simulink model "gm_spectrum_analyser"  (R2020a)
settings: Solver=VariableStepAuto  StartTime=0.0  StopTime=100000/256e6  RelTol=1e-3
InitFcn:
  | fs = 256e6;
undefined symbols (not defined in the file or in its folder): designMultirateFIR
libraries: hdlsllib x81, simulink x50, dspmlti4 x6, dsphdlxfrm x5, hdlmdlgenlib x4, dspswit3 x4, dspsigops x2, dspsigattribs x2
(part 3 of 5)

== system gm_spectrum_analyser/Spectrum Analyser/Spectrum Analyser/Spectrum Analyser Core/FFT and Spectrum Processing/FFT Core ==
  Data In : Inport  OutDataTypeStr=fixdt(1, 16, 15)  PortDimensions=1  SampleTime=3.90625e-09
      settings: SignalType=complex
  Valid In : Inport  Port=2  OutDataTypeStr=boolean  PortDimensions=1  SampleTime=3.90625e-09
  Selector : Inport  Port=3  OutDataTypeStr=uint8  PortDimensions=1  SampleTime=3.90625e-09
  AND{1..5} (5 alike) : Logic  AllPortsSameDT=off  OutDataTypeStr=boolean  SampleTime=3.90625e-09
  Compare To Constant : simulink/Logic and Bit Operations/Compare To Constant  relop===  const="fi(0,0,8,0,\"hex\",\"00\")"  OutDataTypeStr=boolean
  Compare To Constant1 : simulink/Logic and Bit Operations/Compare To Constant  relop===  const="fi(0,0,8,0,\"hex\",\"01\")"  OutDataTypeStr=boolean
  Compare To Constant2 : simulink/Logic and Bit Operations/Compare To Constant  relop===  const="fi(0,0,8,0,\"hex\",\"02\")"  OutDataTypeStr=boolean
  Compare To Constant3 : simulink/Logic and Bit Operations/Compare To Constant  relop===  const="fi(0,0,8,0,\"hex\",\"03\")"  OutDataTypeStr=boolean
  Compare To Constant4 : simulink/Logic and Bit Operations/Compare To Constant  relop===  const="fi(0,0,8,0,\"hex\",\"04\")"  OutDataTypeStr=boolean
  FFT HDL Optimized 16384 : dsphdlxfrm/FFT HDL Optimized  FFTLength=16384  Architecture=Streaming Radix 2^2  ComplexMultiplication=Use 4 multipliers and 2 adders  BitReversedOutput=off  BitReversedInput=off  Normalize=off  SimulateUsing=Code generation  RoundingMethod=Round  ResetInputPort=off  StartOutputPort=on  EndOutputPort=on
      settings: SourceProductBaseCode=DS
  FFT HDL Optimized 32768 : dsphdlxfrm/FFT HDL Optimized  FFTLength=32768  Architecture=Streaming Radix 2^2  ComplexMultiplication=Use 4 multipliers and 2 adders  BitReversedOutput=off  BitReversedInput=off  Normalize=off  SimulateUsing=Code generation  RoundingMethod=Round  ResetInputPort=off  StartOutputPort=on  EndOutputPort=on
      settings: SourceProductBaseCode=DS
  FFT HDL Optimized 4096 : dsphdlxfrm/FFT HDL Optimized  FFTLength=4096  Architecture=Streaming Radix 2^2  ComplexMultiplication=Use 4 multipliers and 2 adders  BitReversedOutput=off  BitReversedInput=off  Normalize=off  SimulateUsing=Code generation  RoundingMethod=Round  ResetInputPort=off  StartOutputPort=on  EndOutputPort=on
      settings: SourceProductBaseCode=DS
  FFT HDL Optimized 65536 : dsphdlxfrm/FFT HDL Optimized  FFTLength=65536  Architecture=Streaming Radix 2^2  ComplexMultiplication=Use 4 multipliers and 2 adders  BitReversedOutput=off  BitReversedInput=off  Normalize=off  SimulateUsing=Code generation  RoundingMethod=Round  ResetInputPort=off  StartOutputPort=on  EndOutputPort=on
      settings: SourceProductBaseCode=DS
  FFT HDL Optimized 8192 : dsphdlxfrm/FFT HDL Optimized  FFTLength=8192  Architecture=Streaming Radix 2^2  ComplexMultiplication=Use 4 multipliers and 2 adders  BitReversedOutput=off  BitReversedInput=off  Normalize=off  SimulateUsing=Code generation  RoundingMethod=Round  ResetInputPort=off  StartOutputPort=on  EndOutputPort=on
      settings: SourceProductBaseCode=DS
  Multiport Switch : MultiPortSwitch  DataPortOrder=Zero-based contiguous  Inputs=5  DiagnosticForDefault=None  zeroidx=on  OutDataTypeStr=fixdt(1, 32, 15)  SampleTime=3.90625e-09
  Multiport Switch1 : MultiPortSwitch  DataPortOrder=Zero-based contiguous  Inputs=5  DiagnosticForDefault=None  zeroidx=on  SampleTime=3.90625e-09
  Multiport Switch2 : MultiPortSwitch  DataPortOrder=Zero-based contiguous  Inputs=5  DiagnosticForDefault=None  zeroidx=on  SampleTime=3.90625e-09
  Multiport Switch3 : MultiPortSwitch  DataPortOrder=Zero-based contiguous  Inputs=5  DiagnosticForDefault=None  zeroidx=on  SampleTime=3.90625e-09
  Data Out : Outport
  Start : Outport  Port=2
  End : Outport  Port=3
  Valid Out : Outport  Port=4
  wires:
  AND1/1 -> FFT HDL Optimized 4096/2
  AND2/1 -> FFT HDL Optimized 8192/2
  AND3/1 -> FFT HDL Optimized 16384/2
  AND4/1 -> FFT HDL Optimized 32768/2
  AND5/1 -> FFT HDL Optimized 65536/2
  Compare To Constant/1 -> AND1/2
  Compare To Constant1/1 -> AND2/2
  Compare To Constant2/1 -> AND3/2
  Compare To Constant3/1 -> AND4/2
  Compare To Constant4/1 -> AND5/2
  FFT HDL Optimized 16384/1 -> Multiport Switch/4
  FFT HDL Optimized 16384/2 -> Multiport Switch1/4
  FFT HDL Optimized 16384/3 -> Multiport Switch2/4
  FFT HDL Optimized 16384/4 -> Multiport Switch3/4
  FFT HDL Optimized 32768/1 -> Multiport Switch/5
  FFT HDL Optimized 32768/2 -> Multiport Switch1/5
  FFT HDL Optimized 32768/3 -> Multiport Switch2/5
  FFT HDL Optimized 32768/4 -> Multiport Switch3/5
  FFT HDL Optimized 4096/1 -> Multiport Switch/2
  FFT HDL Optimized 4096/2 -> Multiport Switch1/2
  FFT HDL Optimized 4096/3 -> Multiport Switch2/2
  FFT HDL Optimized 4096/4 -> Multiport Switch3/2
  FFT HDL Optimized 65536/1 -> Multiport Switch/6
  FFT HDL Optimized 65536/2 -> Multiport Switch1/6
  FFT HDL Optimized 65536/3 -> Multiport Switch2/6
  FFT HDL Optimized 65536/4 -> Multiport Switch3/6
  FFT HDL Optimized 8192/1 -> Multiport Switch/3
  FFT HDL Optimized 8192/2 -> Multiport Switch1/3
  FFT HDL Optimized 8192/3 -> Multiport Switch2/3
  FFT HDL Optimized 8192/4 -> Multiport Switch3/3
  Multiport Switch/1 -> Data Out/1
  Multiport Switch1/1 -> Start/1
  Multiport Switch2/1 -> End/1
  Multiport Switch3/1 -> Valid Out/1
  Data In/1 -> FFT HDL Optimized 16384/1, FFT HDL Optimized 32768/1, FFT HDL Optimized 4096/1, FFT HDL Optimized 65536/1, FFT HDL Optimized 8192/1
  Valid In/1 -> AND5/1, AND4/1, AND3/1, AND2/1, AND1/1
  Selector/1 -> Multiport Switch3/1, Multiport Switch2/1, Multiport Switch1/1, Multiport Switch/1, Compare To Constant4/1, Compare To Constant3/1, Compare To Constant2/1, Compare To Constant1/1, Compare To Constant/1

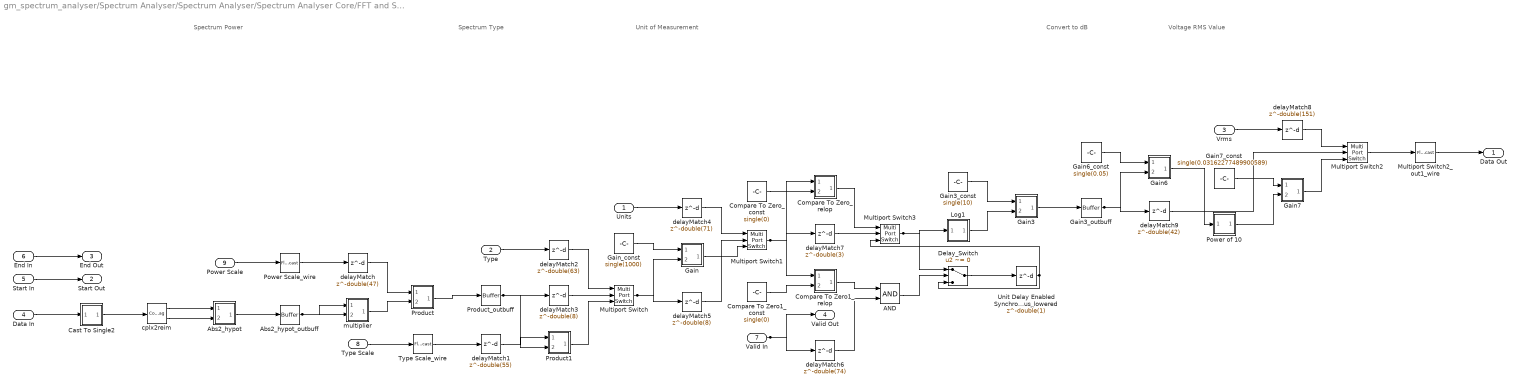
== system gm_spectrum_analyser/Spectrum Analyser/Spectrum Analyser/Spectrum Analyser Core/FFT and Spectrum Processing/Spectrum Options ==
  note: Voltage RMS Value
  note: Convert to dB
  note: Unit of Measurement
  note: Spectrum Type
  note: Spectrum Power
  Units : Inport  OutDataTypeStr=uint32  PortDimensions=1  SampleTime=3.90625e-09
  Type : Inport  Port=2  OutDataTypeStr=uint32  PortDimensions=1  SampleTime=3.90625e-09
  Vrms : Inport  Port=3  OutDataTypeStr=uint32  PortDimensions=1  SampleTime=3.90625e-09
  Data In : Inport  Port=4  OutDataTypeStr=fixdt(1, 32, 15)  PortDimensions=1  SampleTime=3.90625e-09
      settings: SignalType=complex
  Start In : Inport  Port=5  OutDataTypeStr=boolean  PortDimensions=1  SampleTime=3.90625e-09
  End In : Inport  Port=6  OutDataTypeStr=boolean  PortDimensions=1  SampleTime=3.90625e-09
  Valid In : Inport  Port=7  OutDataTypeStr=boolean  PortDimensions=1  SampleTime=3.90625e-09
  Type Scale : Inport  Port=8  OutDataTypeStr=uint32  PortDimensions=1  SampleTime=3.90625e-09
  Power Scale : Inport  Port=9  OutDataTypeStr=uint32  PortDimensions=1  SampleTime=3.90625e-09
  AND : Logic  AllPortsSameDT=off  OutDataTypeStr=boolean  SampleTime=3.90625e-09
  Abs2_hypot : Subsystem
      mask Display: disp('NFP\nmath2');
  Abs2_hypot_outbuff : hdlmdlgenlib/Buffer
      settings: SourceProductBaseCode=SL
  Cast To Single2 : Subsystem
      mask Display: disp('NFP\nconv');
  Compare To Zero1_const : Constant  Value=single(0)  OutDataTypeStr=single  SampleTime=3.90625e-09
  Compare To Zero1_relop : Subsystem
      mask Display: disp('NFP\nrelop');
  Compare To Zero_const : Constant  Value=single(0)  OutDataTypeStr=single  SampleTime=3.90625e-09
  Compare To Zero_relop : Subsystem
      mask Display: disp('NFP\nrelop');
  Delay_Switch : Switch  Criteria=u2 ~= 0  Threshold=double(0)  OutDataTypeStr=single  SampleTime=3.90625e-09
  Gain : Subsystem
      mask Display: disp('NFP\nmul');
  Gain3 : Subsystem
      mask Display: disp('NFP\nmul');
  Gain3_const : Constant  Value=single(10)  OutDataTypeStr=single  SampleTime=3.90625e-09
  Gain3_outbuff : hdlmdlgenlib/Buffer
      settings: SourceProductBaseCode=SL
  Gain6 : Subsystem
      mask Display: disp('NFP\nmul');
  Gain6_const : Constant  Value=single(0.05)  OutDataTypeStr=single  SampleTime=3.90625e-09
  Gain7 : Subsystem
      mask Display: disp('NFP\nmul');
  Gain7_const : Constant  Value=single(0.03162277489900589)  OutDataTypeStr=single  SampleTime=3.90625e-09
  Gain_const : Constant  Value=single(1000)  OutDataTypeStr=single  SampleTime=3.90625e-09
  Log1 : Subsystem
      mask Display: disp('NFP\nmath');
  Multiport Switch{,1..3} (4 alike) : MultiPortSwitch  DataPortOrder=Zero-based contiguous  Inputs=2  DiagnosticForDefault=None  zeroidx=on  OutDataTypeStr=single  SampleTime=3.90625e-09
  Multiport Switch2_out1_wire : FloatTypecast
  Power Scale_wire : FloatTypecast
  Power of 10 : Subsystem
      mask Display: disp('NFP\nmath');
  Product : Subsystem
      mask Display: disp('NFP\nmul');
  Product1 : Subsystem
      mask Display: disp('NFP\nmul');
  Product_outbuff : hdlmdlgenlib/Buffer
      settings: SourceProductBaseCode=SL
  Type Scale_wire : FloatTypecast
  Unit Delay Enabled Synchronous_lowered : Delay  DelayLength=double(1)  InitialCondition=0  SampleTime=3.90625e-09
  cplx2reim : ComplexToRealImag  SampleTime=3.90625e-09
  delayMatch : Delay  DelayLength=double(47)  InitialCondition=0  SampleTime=3.90625e-09
  delayMatch1 : Delay  DelayLength=double(55)  InitialCondition=0  SampleTime=3.90625e-09
  delayMatch2 : Delay  DelayLength=double(63)  InitialCondition=0  SampleTime=3.90625e-09
  delayMatch3 : Delay  DelayLength=double(8)  InitialCondition=0  SampleTime=3.90625e-09
  delayMatch4 : Delay  DelayLength=double(71)  InitialCondition=0  SampleTime=3.90625e-09
  delayMatch5 : Delay  DelayLength=double(8)  InitialCondition=0  SampleTime=3.90625e-09
  delayMatch6 : Delay  DelayLength=double(74)  InitialCondition=0  SampleTime=3.90625e-09
  delayMatch7 : Delay  DelayLength=double(3)  InitialCondition=0  SampleTime=3.90625e-09
  delayMatch8 : Delay  DelayLength=double(151)  InitialCondition=0  SampleTime=3.90625e-09
  delayMatch9 : Delay  DelayLength=double(42)  InitialCondition=0  SampleTime=3.90625e-09
  multiplier : Subsystem
      mask Display: disp('NFP\nmul');
  Data Out : Outport
  Start Out : Outport  Port=2
  End Out : Outport  Port=3
  Valid Out : Outport  Port=4
  wires:
  AND/1 -> Delay_Switch/2
  Abs2_hypot_outbuff/1 -> multiplier/2(In2), multiplier/1(In1)
  Multiport Switch2_out1_wire/1 -> Data Out/1
  delayMatch1/1 -> Product1/1(In1)
  delayMatch/1 -> Product/1(In1)
  delayMatch9/1 -> Multiport Switch2/2
  delayMatch5/1 -> Multiport Switch1/2
  delayMatch7/1 -> Multiport Switch3/2
  Multiport Switch2/1 -> Multiport Switch2_out1_wire/1
  delayMatch3/1 -> Multiport Switch/2
  cplx2reim/1 -> Abs2_hypot/1(In1)
  cplx2reim/2 -> Abs2_hypot/2(In2)
  Compare To Zero_const/1 -> Compare To Zero_relop/2(In2)
  Compare To Zero1_const/1 -> Compare To Zero1_relop/2(In2)
  Gain_const/1 -> Gain/1(In1)
  Gain3_const/1 -> Gain3/1(In1)
  Gain6_const/1 -> Gain6/1(In1)
  Gain7_const/1 -> Gain7/1(In1)
  delayMatch4/1 -> Multiport Switch1/1
  delayMatch2/1 -> Multiport Switch/1
  delayMatch8/1 -> Multiport Switch2/1
  delayMatch6/1 -> AND/2
  Abs2_hypot/1(Out1) -> Abs2_hypot_outbuff/1
  Cast To Single2/1(Out1) -> cplx2reim/1
  Compare To Zero_relop/1(Out1) -> Multiport Switch3/1
  Compare To Zero1_relop/1(Out1) -> AND/1
  Log1/1(Out1) -> Gain3/2(In2)
  Power of 10/1(Out1) -> Gain7/2(In2)
  Product/1(Out1) -> Product_outbuff/1
  Product1/1(Out1) -> Multiport Switch/3
  multiplier/1(Out1) -> Product/2(In2)
  Gain/1(Out1) -> Multiport Switch1/3
  Gain3/1(Out1) -> Gain3_outbuff/1
  Gain6/1(Out1) -> Power of 10/1(In1)
  Gain7/1(Out1) -> Multiport Switch2/3
  Power Scale_wire/1 -> delayMatch/1
  Type Scale_wire/1 -> delayMatch1/1
  Product_outbuff/1 -> delayMatch3/1, Product1/2(In2)
  Multiport Switch/1 -> delayMatch5/1, Gain/2(In2)
  Multiport Switch1/1 -> delayMatch7/1, Compare To Zero1_relop/1(In1), Compare To Zero_relop/1(In1)
  Gain3_outbuff/1 -> delayMatch9/1, Gain6/2(In2)
  Multiport Switch3/1 -> Log1/1(In1), Delay_Switch/1
  Units/1 -> delayMatch4/1
  Type/1 -> delayMatch2/1
  Vrms/1 -> delayMatch8/1
  Data In/1 -> Cast To Single2/1(In1)
  Start In/1 -> Start Out/1
  End In/1 -> End Out/1
  Valid In/1 -> delayMatch6/1, Valid Out/1
  Type Scale/1 -> Type Scale_wire/1
  Power Scale/1 -> Power Scale_wire/1
  Delay_Switch/1 -> Unit Delay Enabled Synchronous_lowered/1
  Unit Delay Enabled Synchronous_lowered/1 -> Multiport Switch3/3, Delay_Switch/3

== system gm_spectrum_analyser/Spectrum Analyser/Spectrum Analyser/Spectrum Analyser Core/Preprocessing Window/Direct Memory Access ==
  axim_rd_s2m : Inport  SampleTime=3.90625e-09
  axim_rd_data : Inport  Port=2  OutDataTypeStr=uint16  PortDimensions=1  SampleTime=3.90625e-09
  Length : Inport  Port=3  OutDataTypeStr=uint32  PortDimensions=1  SampleTime=3.90625e-09
  Address : Inport  Port=4  OutDataTypeStr=uint32  PortDimensions=1  SampleTime=3.90625e-09
  Enable DMA : Inport  Port=5  OutDataTypeStr=uint32  PortDimensions=1  SampleTime=3.90625e-09
  Bit Slice : hdlsllib/Logic and Bit Operations/Bit Slice  lidx=double(0)  ridx=double(0)
      settings: SourceProductBaseCode=SL
  Bus Creator : BusCreator  Inputs=3
  DDR Read Controller : Subsystem
  EdgeDetection : Subsystem
  bus_selector : BusSelector  OutputSignals=rd_aready,rd_dvalid
  ram_wr_data : Outport  VectorParamsAs1DForOutWhenUnconnected=off
  ram_wr_addr : Outport  Port=2  VectorParamsAs1DForOutWhenUnconnected=off
  ram_wren : Outport  Port=3  VectorParamsAs1DForOutWhenUnconnected=off
  dma_read_ready : Outport  Port=4  VectorParamsAs1DForOutWhenUnconnected=off
  axim_rd_m2s : Outport  Port=5  VectorParamsAs1DForOutWhenUnconnected=off
  wires:
  Bit Slice/1 -> EdgeDetection/1(In1)
  Bus Creator/1 -> axim_rd_m2s/1
  bus_selector/1 -> DDR Read Controller/4(rd_aready)  "<rd_aready>"
  bus_selector/2 -> DDR Read Controller/5(rd_dvalid)  "<rd_dvalid>"
  DDR Read Controller/1(valid_out) -> ram_wren/1
  DDR Read Controller/2(count_out) -> ram_wr_addr/1
  DDR Read Controller/3(ready_out) -> dma_read_ready/1
  DDR Read Controller/4(rd_addr) -> Bus Creator/1  "rd_addr"
  DDR Read Controller/5(rd_len) -> Bus Creator/2  "rd_len"
  DDR Read Controller/6(rd_avalid) -> Bus Creator/3  "rd_avalid"
  EdgeDetection/1(Out1) -> DDR Read Controller/3(start)
  axim_rd_s2m/1 -> bus_selector/1
  axim_rd_data/1 -> ram_wr_data/1
  Length/1 -> DDR Read Controller/1(length_in)
  Address/1 -> DDR Read Controller/2(address)
  Enable DMA/1 -> Bit Slice/1

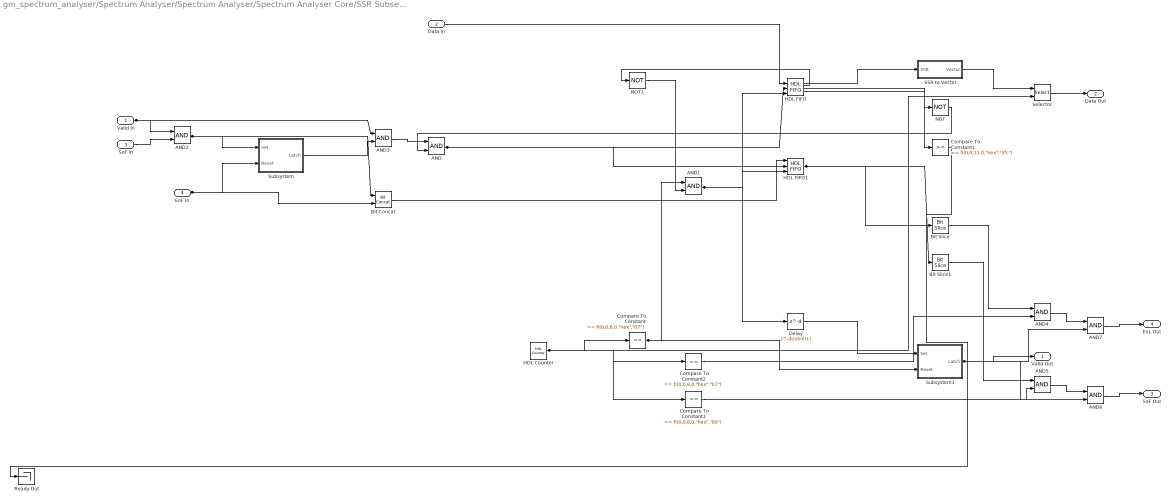
== system gm_spectrum_analyser/Spectrum Analyser/Spectrum Analyser/Spectrum Analyser Core/SSR Subset Converter/SSR Deserializer Imag ==
  Valid In : Inport  OutDataTypeStr=boolean  PortDimensions=1  SampleTime=3.90625e-09
  Data In : Inport  Port=2  OutDataTypeStr=fixdt(0, 128, 0)  PortDimensions=1  SampleTime=3.90625e-09
  SoF In : Inport  Port=3  OutDataTypeStr=boolean  PortDimensions=1  SampleTime=3.90625e-09
  EoF In : Inport  Port=4  OutDataTypeStr=boolean  PortDimensions=1  SampleTime=3.90625e-09
  AND{,1..7} (8 alike) : Logic  AllPortsSameDT=off  OutDataTypeStr=boolean  SampleTime=3.90625e-09
  Bit Concat : hdlsllib/Logic and Bit Operations/Bit Concat  numInputs=2
  Bit Slice : hdlsllib/Logic and Bit Operations/Bit Slice  lidx=double(0)  ridx=double(0)
      settings: SourceProductBaseCode=SL
  Bit Slice1 : hdlsllib/Logic and Bit Operations/Bit Slice  lidx=double(1)  ridx=double(1)
      settings: SourceProductBaseCode=SL
  Compare To Constant : simulink/Logic and Bit Operations/Compare To Constant  relop===  const="fi(0,0,8,0,\"hex\",\"07\")"  OutDataTypeStr=boolean
  Compare To Constant1 : simulink/Logic and Bit Operations/Compare To Constant  relop=>=  const="fi(0,0,11,0,\"hex\",\"3fc\")"  OutDataTypeStr=boolean
  Compare To Constant2 : simulink/Logic and Bit Operations/Compare To Constant  relop===  const="fi(0,0,8,0,\"hex\",\"07\")"  OutDataTypeStr=boolean
  Compare To Constant3 : simulink/Logic and Bit Operations/Compare To Constant  relop===  const="fi(0,0,8,0,\"hex\",\"00\")"  OutDataTypeStr=boolean
  Delay : Delay  DelayLength=double(1)  InitialCondition=0  SampleTime=3.90625e-09
  HDL Counter : hdlsllib/Sources/HDL Counter  CountType=Count limited  CountInit=double(0)  CountStep=double(1)  CountMax=double(7)  CountFromType=Initial value  CountFrom=double(0)  CountResetPort=off  CountLoadPort=off  CountEnbPort=off  CountDirPort=off  CountDataType=Unsigned  CountWordLen=8  CountFracLen=0  CountSampTime=3.90625e-09
  HDL FIFO : hdlsllib/HDL RAMs/HDL FIFO  fifo_size=1024  mode=Classic  ratio=1  push_msg=Error  pop_msg=Error  show_empty=on  show_full=on  show_num=on  LabelModeActiveChoice_Mode=Classic
      settings: SourceProductBaseCode=SL
  HDL FIFO1 : hdlsllib/HDL RAMs/HDL FIFO  fifo_size=1024  mode=Classic  ratio=1  push_msg=Error  pop_msg=Error  show_empty=off  show_full=off  show_num=off  LabelModeActiveChoice_Mode=Classic
      settings: SourceProductBaseCode=SL
  NOT : Logic  Operator=NOT  Inputs=1  AllPortsSameDT=off  OutDataTypeStr=boolean  SampleTime=3.90625e-09
  NOT1 : Logic  Operator=NOT  Inputs=1  AllPortsSameDT=off  OutDataTypeStr=boolean  SampleTime=3.90625e-09
  Ready Out : Terminator
  SSR to Vector : Subsystem  mask{N=double(8), w=double(16), hN=8, hw=16}
      mask prompts: N "Samples per clock cycle:"; w "Wordlength:"
  Selector : Selector  IndexMode=Zero-based  SampleTime=3.90625e-09  IndexOptions=Index vector (port)  Indices=double([1 3])  OutputSizes=double(1)
  Subsystem : Subsystem
  Subsystem1 : Subsystem
  Valid Out : Outport
  Data Out : Outport  Port=2
  SoF Out : Outport  Port=3
  EoL Out : Outport  Port=4
  wires:
  AND/1 -> HDL FIFO1/2, HDL FIFO/2
  AND1/1 -> Delay/1, HDL FIFO1/3, HDL FIFO/3
  AND2/1 -> Bit Concat/1, Subsystem/1(Set)
  AND3/1 -> AND/1
  AND4/1 -> AND7/1
  AND5/1 -> AND6/1
  AND6/1 -> SoF Out/1
  AND7/1 -> EoL Out/1
  Bit Concat/1 -> HDL FIFO1/1
  Bit Slice/1 -> AND4/1
  Bit Slice1/1 -> AND5/1
  Compare To Constant/1 -> Subsystem1/2(Reset), AND1/1
  Compare To Constant1/1 -> Ready Out/1
  Compare To Constant2/1 -> AND4/2
  Compare To Constant3/1 -> AND5/2
  Delay/1 -> Subsystem1/1(Set)
  HDL Counter/1 -> Selector/2, Compare To Constant3/1, Compare To Constant2/1, Compare To Constant/1
  HDL FIFO/1 -> SSR to Vector/1(SSR)
  HDL FIFO/4 -> Compare To Constant1/1
  HDL FIFO1/1 -> Bit Slice1/1, Bit Slice/1
  SSR to Vector/1(Vector) -> Selector/1
  Selector/1 -> Data Out/1
  Subsystem/1(Latch) -> AND3/2
  Subsystem1/1(Latch) -> AND7/2, AND6/2, Valid Out/1
  Valid In/1 -> AND3/1, AND2/1
  Data In/1 -> HDL FIFO/1
  SoF In/1 -> AND2/2
  EoF In/1 -> Bit Concat/2, Subsystem/2(Reset)
  NOT/1 -> AND/2
  HDL FIFO/2 -> NOT1/1
  HDL FIFO/3 -> NOT/1
  NOT1/1 -> AND1/2

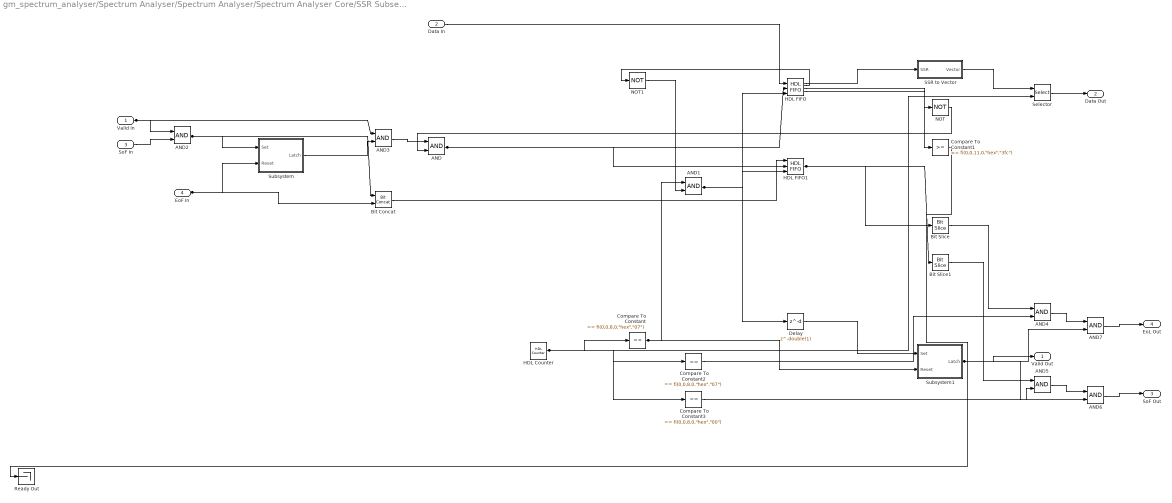
== system gm_spectrum_analyser/Spectrum Analyser/Spectrum Analyser/Spectrum Analyser Core/SSR Subset Converter/SSR Deserializer Real ==
  Valid In : Inport  OutDataTypeStr=boolean  PortDimensions=1  SampleTime=3.90625e-09
  Data In : Inport  Port=2  OutDataTypeStr=fixdt(0, 128, 0)  PortDimensions=1  SampleTime=3.90625e-09
  SoF In : Inport  Port=3  OutDataTypeStr=boolean  PortDimensions=1  SampleTime=3.90625e-09
  EoF In : Inport  Port=4  OutDataTypeStr=boolean  PortDimensions=1  SampleTime=3.90625e-09
  AND{,1..7} (8 alike) : Logic  AllPortsSameDT=off  OutDataTypeStr=boolean  SampleTime=3.90625e-09
  Bit Concat : hdlsllib/Logic and Bit Operations/Bit Concat  numInputs=2
  Bit Slice : hdlsllib/Logic and Bit Operations/Bit Slice  lidx=double(0)  ridx=double(0)
      settings: SourceProductBaseCode=SL
  Bit Slice1 : hdlsllib/Logic and Bit Operations/Bit Slice  lidx=double(1)  ridx=double(1)
      settings: SourceProductBaseCode=SL
  Compare To Constant : simulink/Logic and Bit Operations/Compare To Constant  relop===  const="fi(0,0,8,0,\"hex\",\"07\")"  OutDataTypeStr=boolean
  Compare To Constant1 : simulink/Logic and Bit Operations/Compare To Constant  relop=>=  const="fi(0,0,11,0,\"hex\",\"3fc\")"  OutDataTypeStr=boolean
  Compare To Constant2 : simulink/Logic and Bit Operations/Compare To Constant  relop===  const="fi(0,0,8,0,\"hex\",\"07\")"  OutDataTypeStr=boolean
  Compare To Constant3 : simulink/Logic and Bit Operations/Compare To Constant  relop===  const="fi(0,0,8,0,\"hex\",\"00\")"  OutDataTypeStr=boolean
  Delay : Delay  DelayLength=double(1)  InitialCondition=0  SampleTime=3.90625e-09
  HDL Counter : hdlsllib/Sources/HDL Counter  CountType=Count limited  CountInit=double(0)  CountStep=double(1)  CountMax=double(7)  CountFromType=Initial value  CountFrom=double(0)  CountResetPort=off  CountLoadPort=off  CountEnbPort=off  CountDirPort=off  CountDataType=Unsigned  CountWordLen=8  CountFracLen=0  CountSampTime=3.90625e-09
  HDL FIFO : hdlsllib/HDL RAMs/HDL FIFO  fifo_size=1024  mode=Classic  ratio=1  push_msg=Error  pop_msg=Error  show_empty=on  show_full=on  show_num=on  LabelModeActiveChoice_Mode=Classic
      settings: SourceProductBaseCode=SL
  HDL FIFO1 : hdlsllib/HDL RAMs/HDL FIFO  fifo_size=1024  mode=Classic  ratio=1  push_msg=Error  pop_msg=Error  show_empty=off  show_full=off  show_num=off  LabelModeActiveChoice_Mode=Classic
      settings: SourceProductBaseCode=SL
  NOT : Logic  Operator=NOT  Inputs=1  AllPortsSameDT=off  OutDataTypeStr=boolean  SampleTime=3.90625e-09
  NOT1 : Logic  Operator=NOT  Inputs=1  AllPortsSameDT=off  OutDataTypeStr=boolean  SampleTime=3.90625e-09
  Ready Out : Terminator
  SSR to Vector : Subsystem  mask{N=double(8), w=double(16), hN=8, hw=16}
      mask prompts: N "Samples per clock cycle:"; w "Wordlength:"
  Selector : Selector  IndexMode=Zero-based  SampleTime=3.90625e-09  IndexOptions=Index vector (port)  Indices=double([1 3])  OutputSizes=double(1)
  Subsystem : Subsystem
  Subsystem1 : Subsystem
  Valid Out : Outport
  Data Out : Outport  Port=2
  SoF Out : Outport  Port=3
  EoL Out : Outport  Port=4
  wires:
  AND/1 -> HDL FIFO1/2, HDL FIFO/2
  AND1/1 -> Delay/1, HDL FIFO1/3, HDL FIFO/3
  AND2/1 -> Bit Concat/1, Subsystem/1(Set)
  AND3/1 -> AND/1
  AND4/1 -> AND7/1
  AND5/1 -> AND6/1
  AND6/1 -> SoF Out/1
  AND7/1 -> EoL Out/1
  Bit Concat/1 -> HDL FIFO1/1
  Bit Slice/1 -> AND4/1
  Bit Slice1/1 -> AND5/1
  Compare To Constant/1 -> Subsystem1/2(Reset), AND1/1
  Compare To Constant1/1 -> Ready Out/1
  Compare To Constant2/1 -> AND4/2
  Compare To Constant3/1 -> AND5/2
  Delay/1 -> Subsystem1/1(Set)
  HDL Counter/1 -> Selector/2, Compare To Constant3/1, Compare To Constant2/1, Compare To Constant/1
  HDL FIFO/1 -> SSR to Vector/1(SSR)
  HDL FIFO/4 -> Compare To Constant1/1
  HDL FIFO1/1 -> Bit Slice1/1, Bit Slice/1
  SSR to Vector/1(Vector) -> Selector/1
  Selector/1 -> Data Out/1
  Subsystem/1(Latch) -> AND3/2
  Subsystem1/1(Latch) -> AND7/2, AND6/2, Valid Out/1
  Valid In/1 -> AND3/1, AND2/1
  Data In/1 -> HDL FIFO/1
  SoF In/1 -> AND2/2
  EoF In/1 -> Bit Concat/2, Subsystem/2(Reset)
  NOT/1 -> AND/2
  HDL FIFO/2 -> NOT1/1
  HDL FIFO/3 -> NOT/1
  NOT1/1 -> AND1/2

== system gm_spectrum_analyser/Spectrum Analyser/Spectrum Analyser/Spectrum Analyser Core/SSR Subset Converter/SSR Packet Generator Imag ==
  Frame Drop : Inport  OutDataTypeStr=fixdt(0, 4, 0)  PortDimensions=1  SampleTime=3.90625e-09
  Valid In : Inport  Port=2  OutDataTypeStr=boolean  PortDimensions=1  SampleTime=3.90625e-09
  Data In : Inport  Port=3  OutDataTypeStr=fixdt(0, 128, 0)  PortDimensions=1  SampleTime=3.90625e-09
  Packet Size : Inport  Port=4  OutDataTypeStr=uint32  PortDimensions=1  SampleTime=3.90625e-09
  Frame Dropper : Subsystem
  TLAST Generator : Subsystem
  Valid Out : Outport
  Data Out : Outport  Port=2
  SoF Out : Outport  Port=3
  EoF Out : Outport  Port=4
  wires:
  Frame Dropper/1(Valid Out) -> Valid Out/1
  Frame Dropper/2(Data Out) -> Data Out/1
  Frame Dropper/3(SoF Out) -> SoF Out/1
  Frame Dropper/4(EoF Out) -> EoF Out/1
  TLAST Generator/1(Valid Out) -> Frame Dropper/1(Valid In)
  TLAST Generator/2(Data Out) -> Frame Dropper/2(Data In)
  TLAST Generator/3(SoF Out) -> Frame Dropper/3(SoF In)
  TLAST Generator/4(EoF Out) -> Frame Dropper/4(EoF In)
  Frame Drop/1 -> Frame Dropper/5(Frame Drop)
  Valid In/1 -> TLAST Generator/1(Valid In)
  Data In/1 -> TLAST Generator/2(Data In)
  Packet Size/1 -> TLAST Generator/3(Packet Size)

== system gm_spectrum_analyser/Spectrum Analyser/Spectrum Analyser/Spectrum Analyser Core/SSR Subset Converter/SSR Packet Generator Real ==
  Frame Drop : Inport  OutDataTypeStr=fixdt(0, 4, 0)  PortDimensions=1  SampleTime=3.90625e-09
  Valid In : Inport  Port=2  OutDataTypeStr=boolean  PortDimensions=1  SampleTime=3.90625e-09
  Data In : Inport  Port=3  OutDataTypeStr=fixdt(0, 128, 0)  PortDimensions=1  SampleTime=3.90625e-09
  Packet Size : Inport  Port=4  OutDataTypeStr=uint32  PortDimensions=1  SampleTime=3.90625e-09
  Frame Dropper : Subsystem
  TLAST Generator : Subsystem
  Valid Out : Outport
  Data Out : Outport  Port=2
  SoF Out : Outport  Port=3
  EoF Out : Outport  Port=4
  wires:
  Frame Dropper/1(Valid Out) -> Valid Out/1
  Frame Dropper/2(Data Out) -> Data Out/1
  Frame Dropper/3(SoF Out) -> SoF Out/1
  Frame Dropper/4(EoF Out) -> EoF Out/1
  TLAST Generator/1(Valid Out) -> Frame Dropper/1(Valid In)
  TLAST Generator/2(Data Out) -> Frame Dropper/2(Data In)
  TLAST Generator/3(SoF Out) -> Frame Dropper/3(SoF In)
  TLAST Generator/4(EoF Out) -> Frame Dropper/4(EoF In)
  Frame Drop/1 -> Frame Dropper/5(Frame Drop)
  Valid In/1 -> TLAST Generator/1(Valid In)
  Data In/1 -> TLAST Generator/2(Data In)
  Packet Size/1 -> TLAST Generator/3(Packet Size)

== system gm_spectrum_analyser/Spectrum Analyser/Spectrum Analyser/Spectrum Analyser Core/SSR Subset Converter/SSR Serializer Imag ==
  SSR Control : Inport  OutDataTypeStr=fixdt(0, 4, 0)  PortDimensions=1  SampleTime=3.90625e-09
  Valid In : Inport  Port=2  OutDataTypeStr=boolean  PortDimensions=1  SampleTime=3.90625e-09
  Data In : Inport  Port=3  OutDataTypeStr=fixdt(0, 128, 0)  PortDimensions=1  SampleTime=3.90625e-09
  Bit Slice : hdlsllib/Logic and Bit Operations/Bit Slice  lidx=double(0)  ridx=double(0)
      settings: SourceProductBaseCode=SL
  Bit Slice1 : hdlsllib/Logic and Bit Operations/Bit Slice  lidx=double(1)  ridx=double(0)
      settings: SourceProductBaseCode=SL
  Delay : Delay  DelayLength=double(1)  InitialCondition=0  SampleTime=3.90625e-09
  Delay_Switch : Switch  Criteria=u2 ~= 0  Threshold=double(0)  OutDataTypeStr=uint16  SampleTime=3.90625e-09
  HDL Counter : hdlsllib/Sources/HDL Counter  CountType=Count limited  CountInit=double(0)  CountStep=double(1)  CountMax=double(7)  CountFromType=Initial value  CountFrom=double(0)  CountResetPort=off  CountLoadPort=off  CountEnbPort=on  CountDirPort=off  CountDataType=Unsigned  CountWordLen=3  CountFracLen=0  CountSampTime=3.90625e-09
  Multiport Switch : MultiPortSwitch  DataPortOrder=Zero-based contiguous  Inputs=4  DiagnosticForDefault=None  zeroidx=on  OutDataTypeStr=uint16  SampleTime=3.90625e-09
  Multiport Switch1 : MultiPortSwitch  DataPortOrder=Zero-based contiguous  Inputs=4  DiagnosticForDefault=None  zeroidx=on  SampleTime=3.90625e-09
  SSR to Vector : Subsystem  mask{N=double(8), w=double(16), hN=8, hw=16}
      mask prompts: N "Samples per clock cycle:"; w "Wordlength:"
  SSR1 to SSR8 : Subsystem
  SSR2 to SSR8 : Subsystem
  SSR4 to SSR8 : Subsystem
  Unit Delay Enabled Synchronous_lowered : Delay  DelayLength=double(1)  InitialCondition=0  SampleTime=3.90625e-09
  Vector to SSR : Subsystem  mask{N=double(8), hN=8}
      mask prompts: N "Samples per clock cycle:"
  Valid Out : Outport
  Data Out : Outport  Port=2
  wires:
  Bit Slice/1 -> SSR4 to SSR8/2(Index)
  Bit Slice1/1 -> SSR2 to SSR8/2(Index)
  Delay/1 -> Valid Out/1
  HDL Counter/1 -> Bit Slice1/1, Bit Slice/1, SSR1 to SSR8/2(Index)
  Multiport Switch/1 -> Delay_Switch/1
  Multiport Switch1/1 -> Delay/1, Delay_Switch/2
  SSR to Vector/1(Vector) -> Multiport Switch/5, SSR1 to SSR8/1(Data In), SSR2 to SSR8/1(Data In), SSR4 to SSR8/1(Data In)
  SSR1 to SSR8/1(Data Out) -> Multiport Switch/2
  SSR1 to SSR8/2(Valid Out) -> Multiport Switch1/2
  SSR2 to SSR8/1(Data Out) -> Multiport Switch/3
  SSR2 to SSR8/2(Valid Out) -> Multiport Switch1/3
  SSR4 to SSR8/1(Data Out) -> Multiport Switch/4
  SSR4 to SSR8/2(Valid Out) -> Multiport Switch1/4
  Unit Delay Enabled Synchronous_lowered/1 -> Vector to SSR/1(Vector), Delay_Switch/3
  Vector to SSR/1(SSR) -> Data Out/1
  SSR Control/1 -> Multiport Switch1/1, Multiport Switch/1
  Valid In/1 -> Multiport Switch1/5, HDL Counter/1, SSR4 to SSR8/3(Valid In), SSR1 to SSR8/3(Valid In), SSR2 to SSR8/3(Valid In)
  Data In/1 -> SSR to Vector/1(SSR)
  Delay_Switch/1 -> Unit Delay Enabled Synchronous_lowered/1

== system gm_spectrum_analyser/Spectrum Analyser/Spectrum Analyser/Spectrum Analyser Core/SSR Subset Converter/SSR Serializer Real ==
  SSR Control : Inport  OutDataTypeStr=fixdt(0, 4, 0)  PortDimensions=1  SampleTime=3.90625e-09
  Valid In : Inport  Port=2  OutDataTypeStr=boolean  PortDimensions=1  SampleTime=3.90625e-09
  Data In : Inport  Port=3  OutDataTypeStr=fixdt(0, 128, 0)  PortDimensions=1  SampleTime=3.90625e-09
  Bit Slice : hdlsllib/Logic and Bit Operations/Bit Slice  lidx=double(0)  ridx=double(0)
      settings: SourceProductBaseCode=SL
  Bit Slice1 : hdlsllib/Logic and Bit Operations/Bit Slice  lidx=double(1)  ridx=double(0)
      settings: SourceProductBaseCode=SL
  Delay : Delay  DelayLength=double(1)  InitialCondition=0  SampleTime=3.90625e-09
  Delay_Switch : Switch  Criteria=u2 ~= 0  Threshold=double(0)  OutDataTypeStr=uint16  SampleTime=3.90625e-09
  HDL Counter : hdlsllib/Sources/HDL Counter  CountType=Count limited  CountInit=double(0)  CountStep=double(1)  CountMax=double(7)  CountFromType=Initial value  CountFrom=double(0)  CountResetPort=off  CountLoadPort=off  CountEnbPort=on  CountDirPort=off  CountDataType=Unsigned  CountWordLen=3  CountFracLen=0  CountSampTime=3.90625e-09
  Multiport Switch : MultiPortSwitch  DataPortOrder=Zero-based contiguous  Inputs=4  DiagnosticForDefault=None  zeroidx=on  OutDataTypeStr=uint16  SampleTime=3.90625e-09
  Multiport Switch1 : MultiPortSwitch  DataPortOrder=Zero-based contiguous  Inputs=4  DiagnosticForDefault=None  zeroidx=on  SampleTime=3.90625e-09
  SSR to Vector : Subsystem  mask{N=double(8), w=double(16), hN=8, hw=16}
      mask prompts: N "Samples per clock cycle:"; w "Wordlength:"
  SSR1 to SSR8 : Subsystem
  SSR2 to SSR8 : Subsystem
  SSR4 to SSR8 : Subsystem
  Unit Delay Enabled Synchronous_lowered : Delay  DelayLength=double(1)  InitialCondition=0  SampleTime=3.90625e-09
  Vector to SSR : Subsystem  mask{N=double(8), hN=8}
      mask prompts: N "Samples per clock cycle:"
  Valid Out : Outport
  Data Out : Outport  Port=2
  wires:
  Bit Slice/1 -> SSR4 to SSR8/2(Index)
  Bit Slice1/1 -> SSR2 to SSR8/2(Index)
  Delay/1 -> Valid Out/1
  HDL Counter/1 -> Bit Slice1/1, Bit Slice/1, SSR1 to SSR8/2(Index)
  Multiport Switch/1 -> Delay_Switch/1
  Multiport Switch1/1 -> Delay/1, Delay_Switch/2
  SSR to Vector/1(Vector) -> Multiport Switch/5, SSR4 to SSR8/1(Data In), SSR2 to SSR8/1(Data In), SSR1 to SSR8/1(Data In)
  SSR1 to SSR8/1(Data Out) -> Multiport Switch/2
  SSR1 to SSR8/2(Valid Out) -> Multiport Switch1/2
  SSR2 to SSR8/1(Data Out) -> Multiport Switch/3
  SSR2 to SSR8/2(Valid Out) -> Multiport Switch1/3
  SSR4 to SSR8/1(Data Out) -> Multiport Switch/4
  SSR4 to SSR8/2(Valid Out) -> Multiport Switch1/4
  Unit Delay Enabled Synchronous_lowered/1 -> Vector to SSR/1(Vector), Delay_Switch/3
  Vector to SSR/1(SSR) -> Data Out/1
  SSR Control/1 -> Multiport Switch1/1, Multiport Switch/1
  Valid In/1 -> Multiport Switch1/5, HDL Counter/1, SSR2 to SSR8/3(Valid In), SSR1 to SSR8/3(Valid In), SSR4 to SSR8/3(Valid In)
  Data In/1 -> SSR to Vector/1(SSR)
  Delay_Switch/1 -> Unit Delay Enabled Synchronous_lowered/1

== system gm_spectrum_analyser/Stimulus and Channel/Channel/RF-ADC/NCO and Mixer/RF-ADC Coarse Mixer ==
  Data In : Inport
  Constant : Constant  Value=mc  OutDataTypeStr=fixdt(0,2,0)  SampleTime=-1
  Data Type Conversion : DataTypeConversion  OutDataTypeStr=fixdt(1,16,15)
  Multiport Switch1 : MultiPortSwitch  DataPortOrder=Zero-based contiguous  zeroidx=on
  Negate : Subsystem
  fs_2 : Subsystem
  fs_4 : Subsystem
  Data Out : Outport  VectorParamsAs1DForOutWhenUnconnected=off
  wires:
  Multiport Switch1/1 -> Data Type Conversion/1
  fs_2/1(Data Out) -> Multiport Switch1/2
  Constant/1 -> Multiport Switch1/1
  Data In/1 -> fs_4/1(Data In), fs_2/1(Data In)
  Negate/1(Data Out) -> Multiport Switch1/4
  fs_4/1(Data Out) -> Negate/1(Data In), Multiport Switch1/3
  Data Type Conversion/1 -> Data Out/1

== system gm_spectrum_analyser/Stimulus and Channel/Channel/RF-ADC/NCO and Mixer/RF-ADC Fine Mixer ==
  Data In : Inport
  Complex to Real-Imag : ComplexToRealImag
  Constant : Constant  Value=0  SampleTime=-1
  Multiport Switch : MultiPortSwitch  DataPortOrder=Zero-based contiguous  Inputs=2  zeroidx=on
  NCO : dspsigops/NCO  AccIncSrc=Specify via dialog  AccInc=fix((((fc*1e9)*(2^18))/(fs))*2^30)  PhaseOffsetSrc=Specify via dialog  PhaseOffset=fix((((2^18)*fph)/(2*pi))*2^30)  AccumWL=48  HasDither=off  DitherWL=4  PNgeneratorLength=19  HasPhaseQuantizer=on  TableDepth=18  HasOutputPhaseError=off  Formula=Sine and cosine  DataType=Binary point scaling  OutputWL=16  OutputFL=15  CompMethod=Table lookup (no interpolation)  SampleTime=1/(fs)  SamplesPerFrame=ssr  OutputFrames=off
      settings: SourceProductBaseCode=DS
  Product : Product  OutDataTypeStr=fixdt(1,16,15)
  Product1 : Product  OutDataTypeStr=fixdt(1,16,15)
  Real-Imag to Complex : RealImagToComplex
  Real-Imag to Complex1 : RealImagToComplex
  Shift Arithmetic : ArithShift  BitShiftNumber=1  BitShiftDirection=Right
  Shift Arithmetic1 : ArithShift  BitShiftNumber=1  BitShiftDirection=Right
  Data Out : Outport  VectorParamsAs1DForOutWhenUnconnected=off
  wires:
  Data In/1 -> Product1/1, Product/1
  Constant/1 -> Multiport Switch/1
  Multiport Switch/1 -> Data Out/1
  Complex to Real-Imag/2 -> Shift Arithmetic/1
  Complex to Real-Imag/1 -> Shift Arithmetic1/1
  Shift Arithmetic1/1 -> Real-Imag to Complex1/1
  Shift Arithmetic/1 -> Real-Imag to Complex1/2
  Real-Imag to Complex1/1 -> Multiport Switch/3
  NCO/1 -> Product/2
  NCO/2 -> Product1/2
  Real-Imag to Complex/1 -> Multiport Switch/2, Complex to Real-Imag/1
  Product1/1 -> Real-Imag to Complex/1
  Product/1 -> Real-Imag to Complex/2

== system gm_spectrum_analyser/Stimulus and Channel/Channel/RF-ADC/SSR Converter RF-ADC/Vector to SSR Imag ==
  Vector : Inport
  Bit Concat : hdlsllib/Logic and Bit Operations/Bit Concat  numInputs=8
  Selector0 : Selector  InputPortWidth=8  IndexOptions=Index vector (dialog)  Indices=8  OutputSizes=1
  Selector1 : Selector  InputPortWidth=8  IndexOptions=Index vector (dialog)  Indices=7  OutputSizes=1
  Selector2 : Selector  InputPortWidth=8  IndexOptions=Index vector (dialog)  Indices=6  OutputSizes=1
  Selector3 : Selector  InputPortWidth=8  IndexOptions=Index vector (dialog)  Indices=5  OutputSizes=1
  Selector4 : Selector  InputPortWidth=8  IndexOptions=Index vector (dialog)  Indices=4  OutputSizes=1
  Selector5 : Selector  InputPortWidth=8  IndexOptions=Index vector (dialog)  Indices=3  OutputSizes=1
  Selector6 : Selector  InputPortWidth=8  IndexOptions=Index vector (dialog)  Indices=2  OutputSizes=1
  Selector7 : Selector  InputPortWidth=8  IndexOptions=Index vector (dialog)  Indices=1  OutputSizes=1
  SSR : Outport
  wires:
  Selector7/1 -> Bit Concat/8
  Selector6/1 -> Bit Concat/7
  Selector5/1 -> Bit Concat/6
  Selector4/1 -> Bit Concat/5
  Selector3/1 -> Bit Concat/4
  Selector2/1 -> Bit Concat/3
  Selector1/1 -> Bit Concat/2
  Selector0/1 -> Bit Concat/1
  Vector/1 -> Selector7/1, Selector6/1, Selector5/1, Selector4/1, Selector3/1, Selector2/1, Selector1/1, Selector0/1
  Bit Concat/1 -> SSR/1

== system gm_spectrum_analyser/Stimulus and Channel/Channel/RF-ADC/SSR Converter RF-ADC/Vector to SSR Real ==
  Vector : Inport
  Bit Concat : hdlsllib/Logic and Bit Operations/Bit Concat  numInputs=8
  Selector0 : Selector  InputPortWidth=8  IndexOptions=Index vector (dialog)  Indices=8  OutputSizes=1
  Selector1 : Selector  InputPortWidth=8  IndexOptions=Index vector (dialog)  Indices=7  OutputSizes=1
  Selector2 : Selector  InputPortWidth=8  IndexOptions=Index vector (dialog)  Indices=6  OutputSizes=1
  Selector3 : Selector  InputPortWidth=8  IndexOptions=Index vector (dialog)  Indices=5  OutputSizes=1
  Selector4 : Selector  InputPortWidth=8  IndexOptions=Index vector (dialog)  Indices=4  OutputSizes=1
  Selector5 : Selector  InputPortWidth=8  IndexOptions=Index vector (dialog)  Indices=3  OutputSizes=1
  Selector6 : Selector  InputPortWidth=8  IndexOptions=Index vector (dialog)  Indices=2  OutputSizes=1
  Selector7 : Selector  InputPortWidth=8  IndexOptions=Index vector (dialog)  Indices=1  OutputSizes=1
  SSR : Outport
  wires:
  Selector7/1 -> Bit Concat/8
  Selector6/1 -> Bit Concat/7
  Selector5/1 -> Bit Concat/6
  Selector4/1 -> Bit Concat/5
  Selector3/1 -> Bit Concat/4
  Selector2/1 -> Bit Concat/3
  Selector1/1 -> Bit Concat/2
  Selector0/1 -> Bit Concat/1
  Vector/1 -> Selector0/1, Selector1/1, Selector2/1, Selector3/1, Selector4/1, Selector5/1, Selector7/1, Selector6/1
  Bit Concat/1 -> SSR/1

== system gm_spectrum_analyser/Stimulus and Channel/Channel/RF-DAC/NCO and Mixer/RF-DAC Coarse Mixer ==
  Data In : Inport
  Add2 : Sum  OutDataTypeStr=double
  Complex to Real-Imag : ComplexToRealImag
  Constant : Constant  Value=mc  OutDataTypeStr=fixdt(0,2,0)  SampleTime=-1
  Multiport Switch1 : MultiPortSwitch  DataPortOrder=Zero-based contiguous  zeroidx=on
  Negate : Subsystem
  fs_2 : Subsystem
  fs_4 : Subsystem
  Data Out : Outport  VectorParamsAs1DForOutWhenUnconnected=off
  wires:
  fs_4/1(Data Out) -> Multiport Switch1/3, Negate/1(Data In)
  Negate/1(Data Out) -> Multiport Switch1/4
  Data In/1 -> fs_2/1(Data In), fs_4/1(Data In)
  Constant/1 -> Multiport Switch1/1
  fs_2/1(Data Out) -> Multiport Switch1/2
  Multiport Switch1/1 -> Complex to Real-Imag/1
  Complex to Real-Imag/1 -> Add2/1
  Complex to Real-Imag/2 -> Add2/2
  Add2/1 -> Data Out/1

== system gm_spectrum_analyser/Stimulus and Channel/Channel/RF-DAC/NCO and Mixer/RF-DAC Fine Mixer ==
  Data In : Inport
  Add2 : Sum
  Complex to Real-Imag1 : ComplexToRealImag
  Constant : Constant  OutDataTypeStr=boolean  SampleTime=-1
  Multiport Switch : MultiPortSwitch  DataPortOrder=Zero-based contiguous  Inputs=2  zeroidx=on
  NCO : dspsigops/NCO  AccIncSrc=Specify via dialog  AccInc=fix((((fc*1e9)*(2^18))/(fs))*2^30)  PhaseOffsetSrc=Specify via dialog  PhaseOffset=fix((((2^18)*fph)/(2*pi))*2^30)  AccumWL=48  HasDither=off  DitherWL=4  PNgeneratorLength=19  HasPhaseQuantizer=on  TableDepth=18  HasOutputPhaseError=off  Formula=Sine and cosine  DataType=Binary point scaling  OutputWL=16  OutputFL=15  CompMethod=Table lookup (no interpolation)  SampleTime=1/(fs)  SamplesPerFrame=ssr  OutputFrames=off
      settings: SourceProductBaseCode=DS
  Product1 : Product
  Product4 : Product
  Shift Arithmetic1 : ArithShift  BitShiftNumber=1  BitShiftDirection=Right
  Data Out : Outport  VectorParamsAs1DForOutWhenUnconnected=off
  wires:
  Shift Arithmetic1/1 -> Multiport Switch/3
  Add2/1 -> Multiport Switch/2, Shift Arithmetic1/1
  Multiport Switch/1 -> Data Out/1
  Constant/1 -> Multiport Switch/1
  Data In/1 -> Complex to Real-Imag1/1
  Product4/1 -> Add2/1
  NCO/1 -> Product4/2
  Complex to Real-Imag1/2 -> Product4/1
  Product1/1 -> Add2/2
  Complex to Real-Imag1/1 -> Product1/1
  NCO/2 -> Product1/2

== system gm_spectrum_analyser/Stimulus and Channel/Channel/RF-DAC/SSR Converter RF-DAC/SSR to Vector Low ==
  SSR : Inport
  Bit Slice0 : hdlsllib/Logic and Bit Operations/Bit Slice  lidx=31  ridx=0
      settings: SourceProductBaseCode=SL
  Bit Slice1 : hdlsllib/Logic and Bit Operations/Bit Slice  lidx=63  ridx=32
      settings: SourceProductBaseCode=SL
  Bit Slice2 : hdlsllib/Logic and Bit Operations/Bit Slice  lidx=95  ridx=64
      settings: SourceProductBaseCode=SL
  Bit Slice3 : hdlsllib/Logic and Bit Operations/Bit Slice  lidx=127  ridx=96
      settings: SourceProductBaseCode=SL
  Matrix Concatenate : Concatenate  NumInputs=4  Mode=Multidimensional array
  Vector : Outport
  wires:
  Matrix Concatenate/1 -> Vector/1
  SSR/1 -> Bit Slice0/1, Bit Slice1/1, Bit Slice2/1, Bit Slice3/1
  Bit Slice0/1 -> Matrix Concatenate/1
  Bit Slice1/1 -> Matrix Concatenate/2
  Bit Slice2/1 -> Matrix Concatenate/3
  Bit Slice3/1 -> Matrix Concatenate/4

== system gm_spectrum_analyser/Spectrum Analyser/Spectrum Analyser/Direct Memory Access/Direct Memory Access/DDR Communication/Write Controller ==
  valid : Inport  OutDataTypeStr=boolean  PortDimensions=1  SampleTime=3.90625e-09
  count : Inport  Port=2  OutDataTypeStr=uint32  PortDimensions=1  SampleTime=3.90625e-09
  length : Inport  Port=3  OutDataTypeStr=uint32  PortDimensions=1  SampleTime=3.90625e-09
  enable : Inport  Port=4  OutDataTypeStr=boolean  PortDimensions=1  SampleTime=3.90625e-09
  start : Inport  Port=5  OutDataTypeStr=boolean  PortDimensions=1  SampleTime=3.90625e-09
  wr_complete : Inport  Port=6  OutDataTypeStr=boolean  PortDimensions=1  SampleTime=3.90625e-09
  wr_ready : Inport  Port=7  OutDataTypeStr=boolean  PortDimensions=1  SampleTime=3.90625e-09
  empty : Inport  Port=8  OutDataTypeStr=boolean  PortDimensions=1  SampleTime=3.90625e-09
  slib_spectrum_analyser_c2_Write_Controller : MATLAB Function  TreatAsAtomicUnit=on
  push : Outport  VectorParamsAs1DForOutWhenUnconnected=off
  pop : Outport  Port=2
  wr_len : Outport  Port=3  VectorParamsAs1DForOutWhenUnconnected=off
  buffer : Outport  Port=4
  state : Outport  Port=5
  wires:
  slib_spectrum_analyser_c2_Write_Controller/1(push) -> push/1
  slib_spectrum_analyser_c2_Write_Controller/2(pop) -> pop/1
  slib_spectrum_analyser_c2_Write_Controller/3(wr_len) -> wr_len/1
  slib_spectrum_analyser_c2_Write_Controller/4(buffer) -> buffer/1
  slib_spectrum_analyser_c2_Write_Controller/5(state) -> state/1
  valid/1 -> slib_spectrum_analyser_c2_Write_Controller/1(valid)
  count/1 -> slib_spectrum_analyser_c2_Write_Controller/2(count)
  length/1 -> slib_spectrum_analyser_c2_Write_Controller/3(length)
  enable/1 -> slib_spectrum_analyser_c2_Write_Controller/4(enable)
  start/1 -> slib_spectrum_analyser_c2_Write_Controller/5(start)
  wr_complete/1 -> slib_spectrum_analyser_c2_Write_Controller/6(wr_complete)
  wr_ready/1 -> slib_spectrum_analyser_c2_Write_Controller/7(wr_ready)
  empty/1 -> slib_spectrum_analyser_c2_Write_Controller/8(empty)

== system gm_spectrum_analyser/Spectrum Analyser/Spectrum Analyser/Spectrum Analyser Core/FFT and Spectrum Processing/Spectrum Options/Abs2_hypot ==
  In1 : Inport
  In2 : Inport  Port=2
  Abs2_hypot : Math  Operator=hypot  SampleTime=3.90625e-09  SaturateOnIntegerOverflow=on
  Abs2_hypot_pd1 : Delay  DelayLength=33
  Out1 : Outport
  wires:
  In1/1 -> Abs2_hypot/1
  In2/1 -> Abs2_hypot/2
  Abs2_hypot/1 -> Abs2_hypot_pd1/1
  Abs2_hypot_pd1/1 -> Out1/1

== system gm_spectrum_analyser/Spectrum Analyser/Spectrum Analyser/Spectrum Analyser Core/FFT and Spectrum Processing/Spectrum Options/Cast To Single2 ==
  In1 : Inport
  Cast To Single2 : DataTypeConversion  OutDataTypeStr=single  SampleTime=3.90625e-09
  Cast To Single2_pd1 : Delay  DelayLength=6
  Out1 : Outport
  wires:
  In1/1 -> Cast To Single2/1
  Cast To Single2/1 -> Cast To Single2_pd1/1
  Cast To Single2_pd1/1 -> Out1/1

== system gm_spectrum_analyser/Spectrum Analyser/Spectrum Analyser/Spectrum Analyser Core/FFT and Spectrum Processing/Spectrum Options/Compare To Zero1_relop ==
  In1 : Inport
  In2 : Inport  Port=2
  Compare To Zero1_relop : RelationalOperator  Operator=~=  OutDataTypeStr=boolean  SampleTime=3.90625e-09  RndMeth=Nearest  InputSameDT=on
  Compare To Zero1_relop_pd1 : Delay  DelayLength=3
  Out1 : Outport
  wires:
  In1/1 -> Compare To Zero1_relop/1
  In2/1 -> Compare To Zero1_relop/2
  Compare To Zero1_relop/1 -> Compare To Zero1_relop_pd1/1
  Compare To Zero1_relop_pd1/1 -> Out1/1

== system gm_spectrum_analyser/Spectrum Analyser/Spectrum Analyser/Spectrum Analyser Core/FFT and Spectrum Processing/Spectrum Options/Compare To Zero_relop ==
  In1 : Inport
  In2 : Inport  Port=2
  Compare To Zero_relop : RelationalOperator  Operator===  OutDataTypeStr=boolean  SampleTime=3.90625e-09  RndMeth=Nearest  InputSameDT=on
  Compare To Zero_relop_pd1 : Delay  DelayLength=3
  Out1 : Outport
  wires:
  In1/1 -> Compare To Zero_relop/1
  In2/1 -> Compare To Zero_relop/2
  Compare To Zero_relop/1 -> Compare To Zero_relop_pd1/1
  Compare To Zero_relop_pd1/1 -> Out1/1

== system gm_spectrum_analyser/Spectrum Analyser/Spectrum Analyser/Spectrum Analyser Core/FFT and Spectrum Processing/Spectrum Options/Gain ==
  In1 : Inport
  In2 : Inport  Port=2
  Gain : Product  Inputs=**  OutDataTypeStr=single  SampleTime=3.90625e-09
  Gain_pd1 : Delay  DelayLength=8
  Out1 : Outport
  wires:
  In1/1 -> Gain/1
  In2/1 -> Gain/2
  Gain/1 -> Gain_pd1/1
  Gain_pd1/1 -> Out1/1

== system gm_spectrum_analyser/Spectrum Analyser/Spectrum Analyser/Spectrum Analyser Core/FFT and Spectrum Processing/Spectrum Options/Gain3 ==
  In1 : Inport
  In2 : Inport  Port=2
  Gain3 : Product  Inputs=**  OutDataTypeStr=single  SampleTime=3.90625e-09
  Gain3_pd1 : Delay  DelayLength=8
  Out1 : Outport
  wires:
  In1/1 -> Gain3/1
  In2/1 -> Gain3/2
  Gain3/1 -> Gain3_pd1/1
  Gain3_pd1/1 -> Out1/1

== system gm_spectrum_analyser/Spectrum Analyser/Spectrum Analyser/Spectrum Analyser Core/FFT and Spectrum Processing/Spectrum Options/Gain6 ==
  In1 : Inport
  In2 : Inport  Port=2
  Gain6 : Product  Inputs=**  OutDataTypeStr=single  SampleTime=3.90625e-09
  Gain6_pd1 : Delay  DelayLength=8
  Out1 : Outport
  wires:
  In1/1 -> Gain6/1
  In2/1 -> Gain6/2
  Gain6/1 -> Gain6_pd1/1
  Gain6_pd1/1 -> Out1/1

== system gm_spectrum_analyser/Spectrum Analyser/Spectrum Analyser/Spectrum Analyser Core/FFT and Spectrum Processing/Spectrum Options/Gain7 ==
  In1 : Inport
  In2 : Inport  Port=2
  Gain7 : Product  Inputs=**  OutDataTypeStr=single  SampleTime=3.90625e-09
  Gain7_pd1 : Delay  DelayLength=8
  Out1 : Outport
  wires:
  In1/1 -> Gain7/1
  In2/1 -> Gain7/2
  Gain7/1 -> Gain7_pd1/1
  Gain7_pd1/1 -> Out1/1

== system gm_spectrum_analyser/Spectrum Analyser/Spectrum Analyser/Spectrum Analyser Core/FFT and Spectrum Processing/Spectrum Options/Log1 ==
  In1 : Inport
  Log1 : Math  Operator=log10  SampleTime=3.90625e-09  SaturateOnIntegerOverflow=on
  Log1_pd1 : Delay  DelayLength=27
  Out1 : Outport
  wires:
  In1/1 -> Log1/1
  Log1/1 -> Log1_pd1/1
  Log1_pd1/1 -> Out1/1

== system gm_spectrum_analyser/Spectrum Analyser/Spectrum Analyser/Spectrum Analyser Core/FFT and Spectrum Processing/Spectrum Options/Power of 10 ==
  In1 : Inport
  Power of 10 : Math  Operator=10^u  SampleTime=3.90625e-09  SaturateOnIntegerOverflow=on
  Power of 10_pd1 : Delay  DelayLength=26
  Out1 : Outport
  wires:
  In1/1 -> Power of 10/1
  Power of 10/1 -> Power of 10_pd1/1
  Power of 10_pd1/1 -> Out1/1

== system gm_spectrum_analyser/Spectrum Analyser/Spectrum Analyser/Spectrum Analyser Core/FFT and Spectrum Processing/Spectrum Options/Product ==
  In1 : Inport
  In2 : Inport  Port=2
  Product : Product  Inputs=**  OutDataTypeStr=single  SampleTime=3.90625e-09
  Product_pd1 : Delay  DelayLength=8
  Out1 : Outport
  wires:
  In1/1 -> Product/1
  In2/1 -> Product/2
  Product/1 -> Product_pd1/1
  Product_pd1/1 -> Out1/1

== system gm_spectrum_analyser/Spectrum Analyser/Spectrum Analyser/Spectrum Analyser Core/FFT and Spectrum Processing/Spectrum Options/Product1 ==
  In1 : Inport
  In2 : Inport  Port=2
  Product1 : Product  Inputs=**  OutDataTypeStr=single  SampleTime=3.90625e-09
  Product1_pd1 : Delay  DelayLength=8
  Out1 : Outport
  wires:
  In1/1 -> Product1/1
  In2/1 -> Product1/2
  Product1/1 -> Product1_pd1/1
  Product1_pd1/1 -> Out1/1

== system gm_spectrum_analyser/Spectrum Analyser/Spectrum Analyser/Spectrum Analyser Core/FFT and Spectrum Processing/Spectrum Options/multiplier ==
  In1 : Inport
  In2 : Inport  Port=2
  multiplier : Product  Inputs=**  OutDataTypeStr=single  SampleTime=3.90625e-09
  multiplier_pd1 : Delay  DelayLength=8
  Out1 : Outport
  wires:
  In1/1 -> multiplier/1
  In2/1 -> multiplier/2
  multiplier/1 -> multiplier_pd1/1
  multiplier_pd1/1 -> Out1/1
